simulink model "wolnozmienny_dyskretyzacja"  (R2017b)
settings: Solver=FixedStepDiscrete  StartTime=0.0  StopTime=0.0  RelTol=1e-3
undefined symbols (not defined in the file): H, W
libraries: CPOiS_SourcesSinks x8, CPOiS_DataManipulation x3
settings Model: Creator=alis  LastModifiedBy=alis

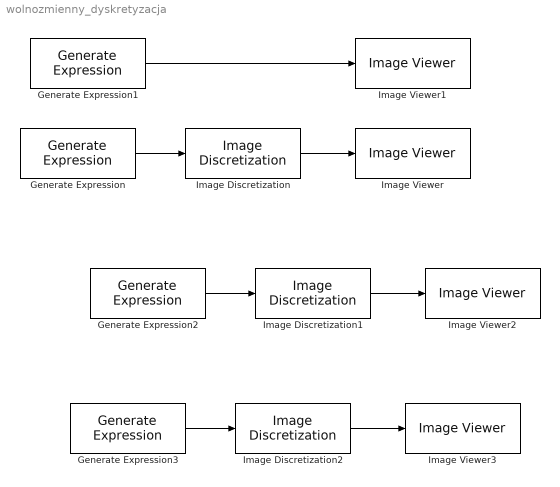
== system wolnozmienny_dyskretyzacja ==
  Generate Expression{,1..3} (4 alike) : CPOiS_SourcesSinks/Generate Expression  Width=256  Height=256  Expression=W/2+H/2
      settings: SourceProductName=CPOiS - Digital image and signal processing
  Image Discretization : CPOiS_DataManipulation/Image Discretization  factor=2
      settings: SourceProductName=CPOiS - Digital image and signal processing
  Image Discretization1 : CPOiS_DataManipulation/Image Discretization  factor=4
      settings: SourceProductName=CPOiS - Digital image and signal processing
  Image Discretization2 : CPOiS_DataManipulation/Image Discretization  factor=8
      settings: SourceProductName=CPOiS - Digital image and signal processing
  Image Viewer{,1..3} (4 alike) : CPOiS_SourcesSinks/Image Viewer
      settings: SourceProductName=CPOiS - Digital image and signal processing
  wires:
  Image Discretization/1 -> Image Viewer/1
  Generate Expression/1 -> Image Discretization/1
  Generate Expression1/1 -> Image Viewer1/1
  Image Discretization1/1 -> Image Viewer2/1
  Generate Expression2/1 -> Image Discretization1/1
  Image Discretization2/1 -> Image Viewer3/1
  Generate Expression3/1 -> Image Discretization2/1
